simulink model "commonlyusedblocks"  (R2016a)
settings: Solver=ode4  StartTime=0.0  StopTime=1  FixedStep=1e-4  RelTol=1e-3
settings Model: Creator=ugurm  LastModifiedBy=mesutto
settings DataIOCC: LimitDataPoints=on  SaveFormat=Array
settings DebuggingCC: UnderspecifiedInitializationDetection=Classic  MergeDetectMultiDrivingBlocksExec=none  SolverPrmCheckMsg=warning  StateNameClashWarn=warning
settings HardwareCC: ProdBitPerPointer=32  ProdLargestAtomicFloat=None  ProdIntDivRoundTo=Undefined  ProdEndianess=Unspecified  ProdWordSize=32  ProdHWDeviceType=32-bit Generic
settings ModelReferenceCC: PropagateSignalLabelsOutOfModel=off
settings ConfigComp: CovModelRefEnable=Off
settings ConfigurationSet: Description=SimMechanics 2G

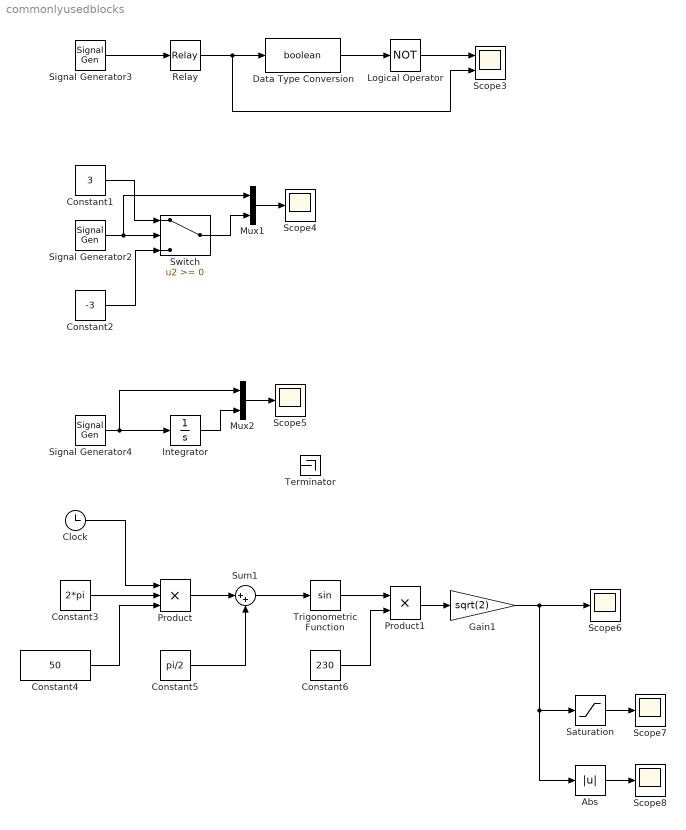
== system commonlyusedblocks ==
  Abs : Abs
  Clock : Clock
  Constant1 : Constant  Value=3
  Constant2 : Constant  Value=-3
  Constant3 : Constant  Value=2*pi
  Constant4 : Constant  Value=50
  Constant5 : Constant  Value=pi/2
  Constant6 : Constant  Value=230
  Data Type Conversion : DataTypeConversion  OutDataTypeStr=boolean
  Gain1 : Gain  Gain=sqrt(2)
  Integrator : Integrator
  Logical Operator : Logic  Operator=NOT  AllPortsSameDT=off  OutDataTypeStr=boolean
  Mux1 : Mux  Inputs=2
  Mux2 : Mux  Inputs=2
  Product : Product  Inputs=3
  Product1 : Product
  Relay : Relay
  Saturation : Saturate  UpperLimit=150  LowerLimit=-150
  Scope3 : Scope  NumInputPorts=2
  Scope{4..8} (5 alike) : Scope
  Signal Generator2 : SignalGenerator  Frequency=50
  Signal Generator3 : SignalGenerator  Frequency=50
  Signal Generator4 : SignalGenerator  WaveForm=square  Frequency=2
  Sum1 : Sum  Inputs=|++
  Switch : Switch
  Terminator : Terminator
  Trigonometric Function : Trigonometry
  wires:
  Relay/1 -> Scope3/2, Data Type Conversion/1
  Data Type Conversion/1 -> Logical Operator/1
  Logical Operator/1 -> Scope3/1
  Signal Generator3/1 -> Relay/1
  Signal Generator2/1 -> Mux1/1, Switch/2
  Constant1/1 -> Switch/1
  Constant2/1 -> Switch/3
  Switch/1 -> Mux1/2
  Mux1/1 -> Scope4/1
  Signal Generator4/1 -> Mux2/1, Integrator/1
  Integrator/1 -> Mux2/2
  Mux2/1 -> Scope5/1
  Constant4/1 -> Product/3
  Constant3/1 -> Product/2
  Clock/1 -> Product/1
  Product/1 -> Sum1/1
  Constant5/1 -> Sum1/2
  Sum1/1 -> Trigonometric Function/1
  Trigonometric Function/1 -> Product1/1
  Product1/1 -> Gain1/1
  Constant6/1 -> Product1/2
  Gain1/1 -> Abs/1, Saturation/1, Scope6/1
  Saturation/1 -> Scope7/1
  Abs/1 -> Scope8/1
